simulink model "gm_Copy_of_uz_pmsm_model_9ph_21b_all_double"  (R2021b)
settings: Solver=FixedStepAuto  StartTime=0.0  StopTime=0.8  RelTol=1e-3
PreLoadFcn:
  | uz_pmsm_model_9ph_init_parameter
undefined symbols (not defined in the file or in its folder): a, b, c, friction_coefficient, inertia, k_i_d, k_i_q, k_p_d, k_p_q, Kpd, L_d, L_o1, L_o2, L_q, L_x1, L_x2, L_y1, L_y2, L_zero, polepair, psi_pm, R_1, static_friction_torque, Tnd, ts
libraries: hdlsllib x90, hdlmdlgenlib x17, slpidlib x2, simulink x2, spsAlphaBetaZerotodq0Lib x1, pid_lib x1, spsdq0toAlphaBetaZeroLib x1
(part 3 of 3)

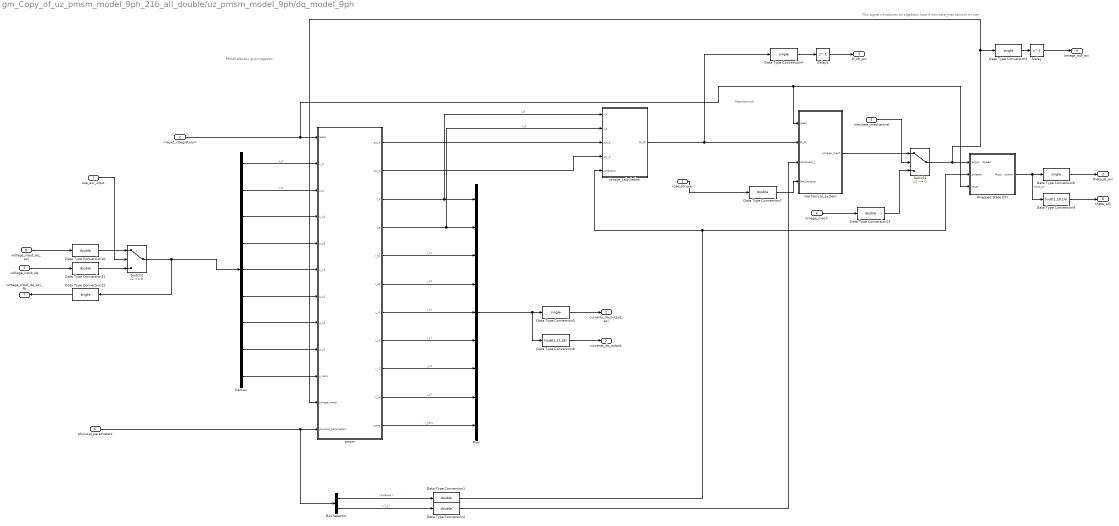
== system gm_Copy_of_uz_pmsm_model_9ph_21b_all_double/uz_pmsm_model_9ph/dq_model_9ph ==
  note: This signal introduces an algebraic loop if simulate_mechanical is true!
  note: PMSM electric and magentic
  note: Mechanical
  load_torque : Inport
  <reset_integrators> : Inport  Port=2
  simulate_mechanical : Inport  Port=3
  omega_mech : Inport  Port=4
  voltage_input_dq : Inport  Port=5
  physical_parameters : Inport  Port=6
  use_axi_input : Inport  Port=7
  voltage_input_dq_axi : Inport  Port=8
  Bus Selector : BusSelector  OutputSignals=polepair,1_J
  Data Type Conversion{1..2,7,10..11,13} (6 alike) : DataTypeConversion  OutDataTypeStr=double  RndMeth=Nearest
  Data Type Conversion{3..6,12} (5 alike) : DataTypeConversion  OutDataTypeStr=single  RndMeth=Nearest
  Data Type Conversion8 : DataTypeConversion  OutDataTypeStr=fixdt(1,27,18)  RndMeth=Nearest
  Data Type Conversion9 : DataTypeConversion  OutDataTypeStr=fixdt(1,18,14)  RndMeth=Nearest
  Delay : Delay  DelayLength=1
  Delay1 : Delay  DelayLength=1
  Demux : Demux  Outputs=9
  Mux : Mux  Inputs=9
  Switch1 : Switch  Criteria=u2 ~= 0
  Switch2 : Switch  Criteria=u2 ~= 0
  Wrapped State DTI : Subsystem
  mechanical_system : Subsystem
  pmsm : Subsystem
  torque_calculation : Subsystem
  currents_dq_output_axi : Outport
  theta_el_axi : Outport  Port=2
  M_Mi_axi : Outport  Port=3
  omega_out_axi : Outport  Port=4
  currents_dq_output : Outport  Port=5
  theta_el1 : Outport  Port=6
  voltage_input_dq_axi_fb : Outport  Port=7
  wires:
  Demux/5 -> pmsm/6(u_x1)
  Demux/7 -> pmsm/8(u_x2)
  Demux/3 -> pmsm/4(u_o1)
  pmsm/3(I_d) -> torque_calculation/1(I_d), Mux/1  "i_d"
  Demux/1 -> pmsm/2(u_d)  "u_d"
  pmsm/11(i_zero) -> Mux/9  "i_zero"
  pmsm/6(i_o2) -> Mux/4  "i_o2"
  Demux/4 -> pmsm/5(u_o2)
  Demux/2 -> pmsm/3(u_q)  "u_q"
  Demux/9 -> pmsm/10(u_zero)
  pmsm/9(i_x2) -> Mux/7  "i_x2"
  pmsm/7(i_x1) -> Mux/5  "i_x1"
  pmsm/10(i_y2) -> Mux/8  "i_y2"
  torque_calculation/1(M_Mi) -> Data Type Conversion4/1, mechanical_system/2(M_Mi)
  Demux/8 -> pmsm/9(u_y2)
  pmsm/1(psi_d) -> torque_calculation/3(psi_d)
  omega_mech/1 -> Data Type Conversion13/1
  pmsm/2(psi_q) -> torque_calculation/4(psi_q)
  simulate_mechanical/1 -> Switch1/2
  Demux/6 -> pmsm/7(u_y1)
  pmsm/5(i_o1) -> Mux/3  "i_o1"
  <reset_integrators>/1 -> Wrapped State DTI/3(reset), mechanical_system/1(reset), pmsm/1(reset)
  pmsm/4(I_q) -> torque_calculation/2(I_q), Mux/2  "i_q"
  mechanical_system/1(omega_mech) -> Switch1/1
  load_torque/1 -> Data Type Conversion7/1
  Switch1/1 -> pmsm/11(omega_mech), Data Type Conversion5/1, Wrapped State DTI/1(Angular Speed)
  pmsm/8(i_y1) -> Mux/6  "i_y1"
  Mux/1 -> Data Type Conversion8/1, Data Type Conversion3/1
  Bus Selector/1 -> Data Type Conversion1/1  "<polepair>"
  Bus Selector/2 -> Data Type Conversion2/1  "<1_J>"
  Delay/1 -> omega_out_axi/1
  Delay1/1 -> M_Mi_axi/1
  Switch2/1 -> Data Type Conversion12/1, Demux/1
  physical_parameters/1 -> Bus Selector/1, pmsm/12(physical_parameters)
  Data Type Conversion1/1 -> torque_calculation/5(polepairs), Wrapped State DTI/2(polepair)
  Data Type Conversion2/1 -> mechanical_system/3(reciprocal_J)
  Data Type Conversion3/1 -> currents_dq_output_axi/1
  Data Type Conversion4/1 -> Delay1/1
  Data Type Conversion5/1 -> Delay/1
  Data Type Conversion6/1 -> theta_el_axi/1
  Wrapped State DTI/1(Angular Position) -> Data Type Conversion9/1, Data Type Conversion6/1  "theta_el"
  Data Type Conversion7/1 -> mechanical_system/4(load_torque)
  Data Type Conversion9/1 -> theta_el1/1
  use_axi_input/1 -> Switch2/2
  voltage_input_dq/1 -> Data Type Conversion11/1
  voltage_input_dq_axi/1 -> Data Type Conversion10/1
  Data Type Conversion10/1 -> Switch2/1
  Data Type Conversion11/1 -> Switch2/3
  Data Type Conversion12/1 -> voltage_input_dq_axi_fb/1
  Data Type Conversion13/1 -> Switch1/3
  Data Type Conversion8/1 -> currents_dq_output/1

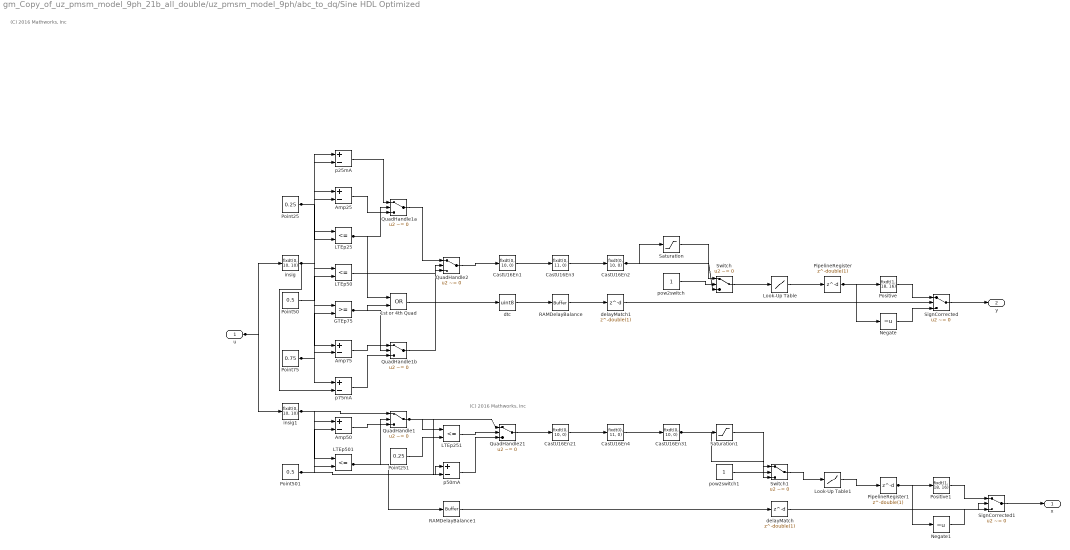
== system gm_Copy_of_uz_pmsm_model_9ph_21b_all_double/uz_pmsm_model_9ph/abc_to_dq/Sine HDL Optimized ==
  note: (C) 2016 Mathworks, Inc
  note: (C) 2016 Mathworks, Inc
  u : Inport  OutDataTypeStr=fixdt(1, 18, 16)  SampleTime=1e-08
  1st or 4th Quad : Logic  Operator=OR  AllPortsSameDT=off  OutDataTypeStr=boolean  SampleTime=1e-08
  Amp25 : Sum  Inputs=+-  AccumDataTypeStr=fixdt(1, 19, 18)  OutDataTypeStr=fixdt(1, 19, 18)  SampleTime=1e-08
  Amp50 : Sum  Inputs=+-  AccumDataTypeStr=fixdt(1, 19, 18)  OutDataTypeStr=fixdt(1, 19, 18)  SampleTime=1e-08
  Amp75 : Sum  Inputs=+-  AccumDataTypeStr=fixdt(1, 19, 18)  OutDataTypeStr=fixdt(1, 19, 18)  SampleTime=1e-08
  CastU16En1 : DataTypeConversion  OutDataTypeStr=fixdt(0, 10, 0)  ConvertRealWorld=Stored Integer (SI)  SampleTime=1e-08
  CastU16En2 : DataTypeConversion  OutDataTypeStr=fixdt(0, 10, 0)  ConvertRealWorld=Stored Integer (SI)  SampleTime=1e-08  SaturateOnIntegerOverflow=on
  CastU16En21 : DataTypeConversion  OutDataTypeStr=fixdt(0, 10, 0)  ConvertRealWorld=Stored Integer (SI)  SampleTime=1e-08
  CastU16En3 : DataTypeConversion  OutDataTypeStr=fixdt(0, 11, 0)  SampleTime=1e-08
  CastU16En31 : DataTypeConversion  OutDataTypeStr=fixdt(0, 10, 0)  ConvertRealWorld=Stored Integer (SI)  SampleTime=1e-08  SaturateOnIntegerOverflow=on
  CastU16En4 : DataTypeConversion  OutDataTypeStr=fixdt(0, 11, 0)  SampleTime=1e-08
  GTEp75 : RelationalOperator  OutDataTypeStr=boolean  SampleTime=1e-08  RndMeth=Nearest
  LTEp{25,50,251,501} (4 alike) : RelationalOperator  Operator=<=  OutDataTypeStr=boolean  SampleTime=1e-08  RndMeth=Nearest
  Look-Up Table : Lookup_n-D  NumberOfTableDimensions=1  BreakpointsForDimension1="fi(\"numerictype\",numerictype(0,10,0),\"fimath\",fimath(\"RoundingMethod\", \"Floor\",\"OverflowAction\", \"Wrap\",\"ProductMode\",\"FullPrecision\",\"SumMode\",\"FullPrecision\"),\"Value\",\"[0 1 2 3 4 5 6 7 8 9 10 11 12 13 14 15 16 17 18 19 20 21 22 23 24 25 26 27 28 29 30 31 32 33 34 35 36 37 38 39 40 41 42 43 44 45 46 47 48 49 50 51 52 53 54 55 56 57 58 59 60 61 62 63 64 65 66 67 68 69 70 71 72 73 74 75 76 77 78 79 80 81 82 83 84 85 86 87 88 89 90 91 92 93 94 95 96 97 98 99 100 101 102 103 104 105 106 107 108 109 110 111 112 113 114 115 116 117 118 119 120 121 122 123 124 125 126 127 128 129 130 131 132 133 134 135 136 137 138 139 140 141 142 143 144 145 146 147 148 149 150 151 152 153 154 155 156 157 158 159 160 161 162 163 164 165 166 167 168 169 170 171 172 173 174 175 176 177 178 179 180 181 182 183 184 185 186 187 188 189 190 191 192 193 194 195 196 197 198 199 200 201 202 203 204 205 206 207 208 209 210 211 212 213 214 215 216 217 218 219 220 221 222 223 224 225 226 227 228 229 230 231 232 233 234 235 236 237 238 239 240 241 242 243 244 245 246 247 248 249 250 251 252 253 254 255]\")"  Table="reshape(fi(\"numerictype\",numerictype(1,18,16),\"fimath\",fimath(\"RoundingMethod\", \"Floor\",\"OverflowAction\", \"Wrap\",\"ProductMode\",\"FullPrecision\",\"SumMode\",\"FullPrecision\"),\"Value\",\"[0;0.006134033203125;0.01226806640625;0.018402099609375;0.0245361328125;0.030670166015625;0.03680419921875;0.042938232421875;0.049072265625;0.0551910400390625;0.0613250732421875;0.06744384765625;0.0735626220703125;0.079681396484375;0.0858001708984375;0.0919036865234375;0.0980224609375;0.1041259765625;0.1102294921875;0.1163177490234375;0.122406005859375;0.1284942626953125;0.13458251953125;0.140655517578125;0.146728515625;0.152801513671875;0.1588592529296875;0.1649169921875;0.17095947265625;0.177001953125;0.18304443359375;0.1890716552734375;0.1950836181640625;0.20111083984375;0.2071075439453125;0.213104248046875;0.2191009521484375;0.2250823974609375;0.2310638427734375;0.237030029296875;0.24298095703125;0.248931884765625;0.2548675537109375;0.2607879638671875;0.2667083740234375;0.2726287841796875;0.2785186767578125;0.2844085693359375;0.290283203125;0.2961578369140625;0.302001953125;0.3078460693359375;0.3136749267578125;0.3195037841796875;0.3253173828125;0.3311004638671875;0.336883544921875;0.3426666259765625;0.348419189453125;0.354156494140625;0.359893798828125;0.3656158447265625;0.3713226318359375;0.37701416015625;0.3826904296875;0.3883514404296875;0.3939971923828125;0.399627685546875;0.405242919921875;0.4108428955078125;0.4164276123046875;0.4219970703125;0.42755126953125;0.4330902099609375;0.4386138916015625;0.444122314453125;0.449615478515625;0.455078125;0.460540771484375;0.465972900390625;0.4713897705078125;0.476806640625;0.482177734375;0.487548828125;0.4929046630859375;0.49822998046875;0.5035400390625;0.5088348388671875;0.51409912109375;0.5193634033203125;0.52459716796875;0.5298004150390625;0.535003662109375;0.5401763916015625;0.545318603515625;0.5504608154296875;0.555572509765625;0.5606689453125;0.56573486328125;0.5707855224609375;0.5758056640625;0.580810546875;0.5858001708984375;0.59075927734375;0.595703125;0.600616455078125;0.6055145263671875;0.610382080078125;0.615234375;0.62005615234375;0.6248626708984375;0.629638671875;0.6343994140625;0.639129638671875;0.643829345703125;0.6485137939453125;0.653167724609375;0.657806396484375;0.66241455078125;0.6670074462890625;0.6715545654296875;0.67608642578125;0.68060302734375;0.685089111328125;0.689544677734375;0.6939697265625;0.6983795166015625;0.7027587890625;0.7071075439453125;0.71142578125;0.715728759765625;0.720001220703125;0.7242431640625;0.7284698486328125;0.7326507568359375;0.73681640625;0.7409515380859375;0.74505615234375;0.7491302490234375;0.7531890869140625;0.7572021484375;0.761199951171875;0.765167236328125;0.76910400390625;0.77301025390625;0.776885986328125;0.780731201171875;0.7845611572265625;0.7883453369140625;0.7920989990234375;0.79583740234375;0.799530029296875;0.8032073974609375;0.806854248046875;0.810455322265625;0.8140411376953125;0.8175811767578125;0.82110595703125;0.8245849609375;0.8280487060546875;0.8314666748046875;0.834869384765625;0.838226318359375;0.841552734375;0.8448486328125;0.848114013671875;0.851348876953125;0.85455322265625;0.85772705078125;0.860870361328125;0.8639678955078125;0.8670501708984375;0.870086669921875;0.8730926513671875;0.876068115234375;0.8790130615234375;0.881927490234375;0.884796142578125;0.88763427734375;0.89044189453125;0.893218994140625;0.895965576171875;0.898681640625;0.9013519287109375;0.90399169921875;0.9066009521484375;0.9091644287109375;0.911712646484375;0.914215087890625;0.9166717529296875;0.9191131591796875;0.9215087890625;0.9238739013671875;0.92620849609375;0.9285125732421875;0.9307708740234375;0.9329986572265625;0.9351806640625;0.9373321533203125;0.939453125;0.9415435791015625;0.9435882568359375;0.9456024169921875;0.9475860595703125;0.94952392578125;0.9514312744140625;0.95330810546875;0.95513916015625;0.956939697265625;0.958709716796875;0.9604339599609375;0.962127685546875;0.963775634765625;0.96539306640625;0.96697998046875;0.9685211181640625;0.97003173828125;0.97149658203125;0.9729461669921875;0.974334716796875;0.9757080078125;0.9770355224609375;0.9783172607421875;0.9795684814453125;0.9807891845703125;0.981964111328125 ...(+541 chars)]\"), [1  256])"  InterpMethod=Flat  ExtrapMethod=Clip  DiagnosticForOutOfRangeInput=Error  SampleTime=1e-08  OutDataTypeStr=fixdt(1, 18, 16)  InputSameDT=on
  Look-Up Table1 : Lookup_n-D  NumberOfTableDimensions=1  BreakpointsForDimension1="fi(\"numerictype\",numerictype(0,10,0),\"fimath\",fimath(\"RoundingMethod\", \"Floor\",\"OverflowAction\", \"Wrap\",\"ProductMode\",\"FullPrecision\",\"SumMode\",\"FullPrecision\"),\"Value\",\"[0 1 2 3 4 5 6 7 8 9 10 11 12 13 14 15 16 17 18 19 20 21 22 23 24 25 26 27 28 29 30 31 32 33 34 35 36 37 38 39 40 41 42 43 44 45 46 47 48 49 50 51 52 53 54 55 56 57 58 59 60 61 62 63 64 65 66 67 68 69 70 71 72 73 74 75 76 77 78 79 80 81 82 83 84 85 86 87 88 89 90 91 92 93 94 95 96 97 98 99 100 101 102 103 104 105 106 107 108 109 110 111 112 113 114 115 116 117 118 119 120 121 122 123 124 125 126 127 128 129 130 131 132 133 134 135 136 137 138 139 140 141 142 143 144 145 146 147 148 149 150 151 152 153 154 155 156 157 158 159 160 161 162 163 164 165 166 167 168 169 170 171 172 173 174 175 176 177 178 179 180 181 182 183 184 185 186 187 188 189 190 191 192 193 194 195 196 197 198 199 200 201 202 203 204 205 206 207 208 209 210 211 212 213 214 215 216 217 218 219 220 221 222 223 224 225 226 227 228 229 230 231 232 233 234 235 236 237 238 239 240 241 242 243 244 245 246 247 248 249 250 251 252 253 254 255]\")"  Table="reshape(fi(\"numerictype\",numerictype(1,18,16),\"fimath\",fimath(\"RoundingMethod\", \"Floor\",\"OverflowAction\", \"Wrap\",\"ProductMode\",\"FullPrecision\",\"SumMode\",\"FullPrecision\"),\"Value\",\"[0;0.006134033203125;0.01226806640625;0.018402099609375;0.0245361328125;0.030670166015625;0.03680419921875;0.042938232421875;0.049072265625;0.0551910400390625;0.0613250732421875;0.06744384765625;0.0735626220703125;0.079681396484375;0.0858001708984375;0.0919036865234375;0.0980224609375;0.1041259765625;0.1102294921875;0.1163177490234375;0.122406005859375;0.1284942626953125;0.13458251953125;0.140655517578125;0.146728515625;0.152801513671875;0.1588592529296875;0.1649169921875;0.17095947265625;0.177001953125;0.18304443359375;0.1890716552734375;0.1950836181640625;0.20111083984375;0.2071075439453125;0.213104248046875;0.2191009521484375;0.2250823974609375;0.2310638427734375;0.237030029296875;0.24298095703125;0.248931884765625;0.2548675537109375;0.2607879638671875;0.2667083740234375;0.2726287841796875;0.2785186767578125;0.2844085693359375;0.290283203125;0.2961578369140625;0.302001953125;0.3078460693359375;0.3136749267578125;0.3195037841796875;0.3253173828125;0.3311004638671875;0.336883544921875;0.3426666259765625;0.348419189453125;0.354156494140625;0.359893798828125;0.3656158447265625;0.3713226318359375;0.37701416015625;0.3826904296875;0.3883514404296875;0.3939971923828125;0.399627685546875;0.405242919921875;0.4108428955078125;0.4164276123046875;0.4219970703125;0.42755126953125;0.4330902099609375;0.4386138916015625;0.444122314453125;0.449615478515625;0.455078125;0.460540771484375;0.465972900390625;0.4713897705078125;0.476806640625;0.482177734375;0.487548828125;0.4929046630859375;0.49822998046875;0.5035400390625;0.5088348388671875;0.51409912109375;0.5193634033203125;0.52459716796875;0.5298004150390625;0.535003662109375;0.5401763916015625;0.545318603515625;0.5504608154296875;0.555572509765625;0.5606689453125;0.56573486328125;0.5707855224609375;0.5758056640625;0.580810546875;0.5858001708984375;0.59075927734375;0.595703125;0.600616455078125;0.6055145263671875;0.610382080078125;0.615234375;0.62005615234375;0.6248626708984375;0.629638671875;0.6343994140625;0.639129638671875;0.643829345703125;0.6485137939453125;0.653167724609375;0.657806396484375;0.66241455078125;0.6670074462890625;0.6715545654296875;0.67608642578125;0.68060302734375;0.685089111328125;0.689544677734375;0.6939697265625;0.6983795166015625;0.7027587890625;0.7071075439453125;0.71142578125;0.715728759765625;0.720001220703125;0.7242431640625;0.7284698486328125;0.7326507568359375;0.73681640625;0.7409515380859375;0.74505615234375;0.7491302490234375;0.7531890869140625;0.7572021484375;0.761199951171875;0.765167236328125;0.76910400390625;0.77301025390625;0.776885986328125;0.780731201171875;0.7845611572265625;0.7883453369140625;0.7920989990234375;0.79583740234375;0.799530029296875;0.8032073974609375;0.806854248046875;0.810455322265625;0.8140411376953125;0.8175811767578125;0.82110595703125;0.8245849609375;0.8280487060546875;0.8314666748046875;0.834869384765625;0.838226318359375;0.841552734375;0.8448486328125;0.848114013671875;0.851348876953125;0.85455322265625;0.85772705078125;0.860870361328125;0.8639678955078125;0.8670501708984375;0.870086669921875;0.8730926513671875;0.876068115234375;0.8790130615234375;0.881927490234375;0.884796142578125;0.88763427734375;0.89044189453125;0.893218994140625;0.895965576171875;0.898681640625;0.9013519287109375;0.90399169921875;0.9066009521484375;0.9091644287109375;0.911712646484375;0.914215087890625;0.9166717529296875;0.9191131591796875;0.9215087890625;0.9238739013671875;0.92620849609375;0.9285125732421875;0.9307708740234375;0.9329986572265625;0.9351806640625;0.9373321533203125;0.939453125;0.9415435791015625;0.9435882568359375;0.9456024169921875;0.9475860595703125;0.94952392578125;0.9514312744140625;0.95330810546875;0.95513916015625;0.956939697265625;0.958709716796875;0.9604339599609375;0.962127685546875;0.963775634765625;0.96539306640625;0.96697998046875;0.9685211181640625;0.97003173828125;0.97149658203125;0.9729461669921875;0.974334716796875;0.9757080078125;0.9770355224609375;0.9783172607421875;0.9795684814453125;0.9807891845703125;0.981964111328125 ...(+541 chars)]\"), [1  256])"  InterpMethod=Flat  ExtrapMethod=Clip  DiagnosticForOutOfRangeInput=Error  SampleTime=1e-08  OutDataTypeStr=fixdt(1, 18, 16)  InputSameDT=on
  Negate : UnaryMinus  SampleTime=1e-08
  Negate1 : UnaryMinus  SampleTime=1e-08
  PipelineRegister : Delay  DelayLength=double(1)  InitialCondition=0  SampleTime=1e-08
  PipelineRegister1 : Delay  DelayLength=double(1)  InitialCondition=0  SampleTime=1e-08
  Point25 : Constant  Value=0.25  OutDataTypeStr=fixdt(0, 18, 18)  SampleTime=1e-08
  Point251 : Constant  Value=0.25  OutDataTypeStr=fixdt(0, 18, 18)  SampleTime=1e-08
  Point50 : Constant  Value=0.5  OutDataTypeStr=fixdt(0, 18, 18)  SampleTime=1e-08
  Point501 : Constant  Value=0.5  OutDataTypeStr=fixdt(0, 18, 18)  SampleTime=1e-08
  Point75 : Constant  Value=0.75  OutDataTypeStr=fixdt(0, 18, 18)  SampleTime=1e-08
  Positive : DataTypeConversion  OutDataTypeStr=fixdt(1, 18, 16)  SampleTime=1e-08
  Positive1 : DataTypeConversion  OutDataTypeStr=fixdt(1, 18, 16)  SampleTime=1e-08
  QuadHandle1 : Switch  Criteria=u2 ~= 0  Threshold=double(0)  OutDataTypeStr=fixdt(1, 19, 18)  SampleTime=1e-08
  QuadHandle1a : Switch  Criteria=u2 ~= 0  Threshold=double(0)  OutDataTypeStr=fixdt(1, 19, 18)  SampleTime=1e-08
  QuadHandle1b : Switch  Criteria=u2 ~= 0  Threshold=double(0)  OutDataTypeStr=fixdt(1, 19, 18)  SampleTime=1e-08
  QuadHandle2 : Switch  Criteria=u2 ~= 0  Threshold=double(0)  OutDataTypeStr=fixdt(0, 10, 10)  SampleTime=1e-08  SaturateOnIntegerOverflow=on
  QuadHandle21 : Switch  Criteria=u2 ~= 0  Threshold=double(0)  OutDataTypeStr=fixdt(0, 10, 10)  SampleTime=1e-08
  RAMDelayBalance : hdlmdlgenlib/Buffer
      settings: SourceProductBaseCode=SL
  RAMDelayBalance1 : hdlmdlgenlib/Buffer
      settings: SourceProductBaseCode=SL
  Saturation : Saturate  UpperLimit="fi(0,0,10,0,\"hex\",\"0ff\")"  LowerLimit="fi(0,0,10,0,\"hex\",\"000\")"  SampleTime=1e-08  OutDataTypeStr=fixdt(0, 10, 0)
  Saturation1 : Saturate  UpperLimit="fi(0,0,10,0,\"hex\",\"0ff\")"  LowerLimit="fi(0,0,10,0,\"hex\",\"000\")"  SampleTime=1e-08  OutDataTypeStr=fixdt(0, 10, 0)
  SignCorrected : Switch  Criteria=u2 ~= 0  Threshold=double(0)  OutDataTypeStr=fixdt(1, 18, 16)  SampleTime=1e-08
  SignCorrected1 : Switch  Criteria=u2 ~= 0  Threshold=double(0)  OutDataTypeStr=fixdt(1, 18, 16)  SampleTime=1e-08
  Switch : Switch  Criteria=u2 ~= 0  Threshold=double(0)  OutDataTypeStr=fixdt(0, 10, 0)  SampleTime=1e-08
  Switch1 : Switch  Criteria=u2 ~= 0  Threshold=double(0)  OutDataTypeStr=fixdt(0, 10, 0)  SampleTime=1e-08
  delayMatch : Delay  DelayLength=double(1)  InitialCondition=0  SampleTime=1e-08
  delayMatch1 : Delay  DelayLength=double(1)  InitialCondition=0  SampleTime=1e-08
  dtc : DataTypeConversion  OutDataTypeStr=uint8  SampleTime=1e-08
  insig : DataTypeConversion  OutDataTypeStr=fixdt(0, 10, 10)  SampleTime=1e-08
  insig1 : DataTypeConversion  OutDataTypeStr=fixdt(0, 10, 10)  SampleTime=1e-08
  p25mA : Sum  Inputs=+-  AccumDataTypeStr=fixdt(1, 19, 18)  OutDataTypeStr=fixdt(1, 19, 18)  SampleTime=1e-08
  p50mA : Sum  Inputs=+-  AccumDataTypeStr=fixdt(1, 20, 18)  OutDataTypeStr=fixdt(1, 20, 18)  SampleTime=1e-08
  p75mA : Sum  Inputs=+-  AccumDataTypeStr=fixdt(1, 19, 18)  OutDataTypeStr=fixdt(1, 19, 18)  SampleTime=1e-08
  pow2switch : Constant  OutDataTypeStr=boolean  SampleTime=1e-08
  pow2switch1 : Constant  OutDataTypeStr=boolean  SampleTime=1e-08
  x : Outport  SampleTime=1e-08
  y : Outport  Port=2  SampleTime=1e-08
  wires:
  dtc/1 -> RAMDelayBalance/1
  Amp25/1 -> QuadHandle1a/3
  Amp75/1 -> QuadHandle1b/1
  CastU16En1/1 -> CastU16En3/1
  CastU16En2/1 -> Switch/3, Saturation/1
  CastU16En3/1 -> CastU16En2/1
  GTEp75/1 -> QuadHandle1b/2, 1st or 4th Quad/2
  LTEp25/1 -> QuadHandle1a/2, 1st or 4th Quad/1
  LTEp50/1 -> QuadHandle2/2
  PipelineRegister/1 -> Positive/1, Negate/1
  Negate/1 -> SignCorrected/3
  Point25/1 -> p25mA/1, LTEp25/2, Amp25/2
  Point50/1 -> LTEp50/2
  Point75/1 -> p75mA/1, GTEp75/2, Amp75/2
  Positive/1 -> SignCorrected/1
  QuadHandle1a/1 -> QuadHandle2/1
  QuadHandle1b/1 -> QuadHandle2/3
  QuadHandle2/1 -> CastU16En1/1
  delayMatch1/1 -> SignCorrected/2
  Saturation/1 -> Switch/1
  SignCorrected/1 -> y/1
  Switch/1 -> Look-Up Table/1
  insig/1 -> p75mA/2, p25mA/2, LTEp50/1, LTEp25/1, GTEp75/1, Amp75/1, Amp25/1
  p25mA/1 -> QuadHandle1a/1
  p75mA/1 -> QuadHandle1b/3
  pow2switch/1 -> Switch/2
  Amp50/1 -> QuadHandle1/3
  CastU16En21/1 -> CastU16En4/1
  CastU16En31/1 -> Switch1/3, Saturation1/1
  CastU16En4/1 -> CastU16En31/1
  LTEp251/1 -> QuadHandle21/2
  LTEp501/1 -> QuadHandle1/2, RAMDelayBalance1/1
  PipelineRegister1/1 -> Positive1/1, Negate1/1
  Negate1/1 -> SignCorrected1/3
  Point251/1 -> LTEp251/2
  Point501/1 -> p50mA/1, LTEp501/2, Amp50/2
  Positive1/1 -> SignCorrected1/1
  QuadHandle1/1 -> p50mA/2, QuadHandle21/1, LTEp251/1
  QuadHandle21/1 -> CastU16En21/1
  delayMatch/1 -> SignCorrected1/2
  Saturation1/1 -> Switch1/1
  SignCorrected1/1 -> x/1
  Switch1/1 -> Look-Up Table1/1
  insig1/1 -> QuadHandle1/1, LTEp501/1, Amp50/1
  p50mA/1 -> QuadHandle21/3
  pow2switch1/1 -> Switch1/2
  1st or 4th Quad/1 -> dtc/1
  RAMDelayBalance1/1 -> delayMatch/1
  RAMDelayBalance/1 -> delayMatch1/1
  u/1 -> insig1/1, insig/1
  Look-Up Table/1 -> PipelineRegister/1
  Look-Up Table1/1 -> PipelineRegister1/1

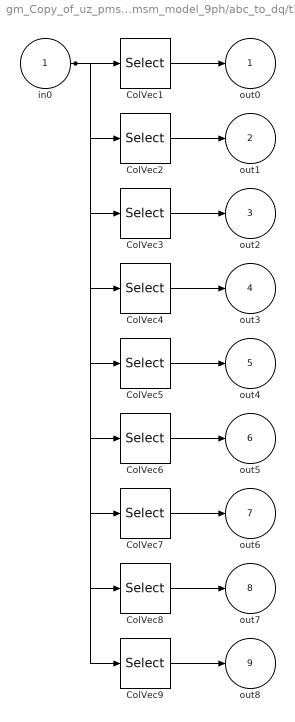
== system gm_Copy_of_uz_pmsm_model_9ph_21b_all_double/uz_pmsm_model_9ph/abc_to_dq/t19 ==
  in0 : Inport
  ColVec1 : Selector  NumberOfDimensions=2  IndexOptions=Select all,Index vector (dialog)  Indices=1,1  OutputSizes=1,1
  ColVec2 : Selector  NumberOfDimensions=2  IndexOptions=Select all,Index vector (dialog)  Indices=1,2  OutputSizes=1,1
  ColVec3 : Selector  NumberOfDimensions=2  IndexOptions=Select all,Index vector (dialog)  Indices=1,3  OutputSizes=1,1
  ColVec4 : Selector  NumberOfDimensions=2  IndexOptions=Select all,Index vector (dialog)  Indices=1,4  OutputSizes=1,1
  ColVec5 : Selector  NumberOfDimensions=2  IndexOptions=Select all,Index vector (dialog)  Indices=1,5  OutputSizes=1,1
  ColVec6 : Selector  NumberOfDimensions=2  IndexOptions=Select all,Index vector (dialog)  Indices=1,6  OutputSizes=1,1
  ColVec7 : Selector  NumberOfDimensions=2  IndexOptions=Select all,Index vector (dialog)  Indices=1,7  OutputSizes=1,1
  ColVec8 : Selector  NumberOfDimensions=2  IndexOptions=Select all,Index vector (dialog)  Indices=1,8  OutputSizes=1,1
  ColVec9 : Selector  NumberOfDimensions=2  IndexOptions=Select all,Index vector (dialog)  Indices=1,9  OutputSizes=1,1
  out0 : Outport
  out1 : Outport  Port=2
  out2 : Outport  Port=3
  out3 : Outport  Port=4
  out4 : Outport  Port=5
  out5 : Outport  Port=6
  out6 : Outport  Port=7
  out7 : Outport  Port=8
  out8 : Outport  Port=9
  wires:
  in0/1 -> ColVec1/1, ColVec2/1, ColVec3/1, ColVec4/1, ColVec5/1, ColVec6/1, ColVec7/1, ColVec8/1, ColVec9/1
  ColVec1/1 -> out0/1
  ColVec2/1 -> out1/1
  ColVec3/1 -> out2/1
  ColVec4/1 -> out3/1
  ColVec5/1 -> out4/1
  ColVec6/1 -> out5/1
  ColVec7/1 -> out6/1
  ColVec8/1 -> out7/1
  ColVec9/1 -> out8/1

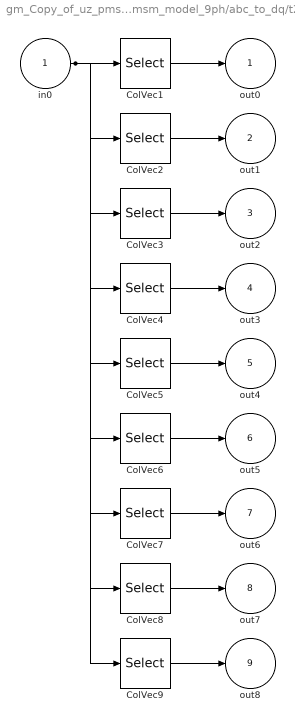
== system gm_Copy_of_uz_pmsm_model_9ph_21b_all_double/uz_pmsm_model_9ph/abc_to_dq/t23 ==
  in0 : Inport
  ColVec1 : Selector  NumberOfDimensions=2  IndexOptions=Select all,Index vector (dialog)  Indices=1,1  OutputSizes=1,1
  ColVec2 : Selector  NumberOfDimensions=2  IndexOptions=Select all,Index vector (dialog)  Indices=1,2  OutputSizes=1,1
  ColVec3 : Selector  NumberOfDimensions=2  IndexOptions=Select all,Index vector (dialog)  Indices=1,3  OutputSizes=1,1
  ColVec4 : Selector  NumberOfDimensions=2  IndexOptions=Select all,Index vector (dialog)  Indices=1,4  OutputSizes=1,1
  ColVec5 : Selector  NumberOfDimensions=2  IndexOptions=Select all,Index vector (dialog)  Indices=1,5  OutputSizes=1,1
  ColVec6 : Selector  NumberOfDimensions=2  IndexOptions=Select all,Index vector (dialog)  Indices=1,6  OutputSizes=1,1
  ColVec7 : Selector  NumberOfDimensions=2  IndexOptions=Select all,Index vector (dialog)  Indices=1,7  OutputSizes=1,1
  ColVec8 : Selector  NumberOfDimensions=2  IndexOptions=Select all,Index vector (dialog)  Indices=1,8  OutputSizes=1,1
  ColVec9 : Selector  NumberOfDimensions=2  IndexOptions=Select all,Index vector (dialog)  Indices=1,9  OutputSizes=1,1
  out0 : Outport
  out1 : Outport  Port=2
  out2 : Outport  Port=3
  out3 : Outport  Port=4
  out4 : Outport  Port=5
  out5 : Outport  Port=6
  out6 : Outport  Port=7
  out7 : Outport  Port=8
  out8 : Outport  Port=9
  wires:
  in0/1 -> ColVec1/1, ColVec2/1, ColVec3/1, ColVec4/1, ColVec5/1, ColVec6/1, ColVec7/1, ColVec8/1, ColVec9/1
  ColVec1/1 -> out0/1
  ColVec2/1 -> out1/1
  ColVec3/1 -> out2/1
  ColVec4/1 -> out3/1
  ColVec5/1 -> out4/1
  ColVec6/1 -> out5/1
  ColVec7/1 -> out6/1
  ColVec8/1 -> out7/1
  ColVec9/1 -> out8/1

== system gm_Copy_of_uz_pmsm_model_9ph_21b_all_double/uz_pmsm_model_9ph/dq_model_9ph/Wrapped State DTI ==
  note: https://de.mathworks.com/help/releases/R2021a/hdlcoder/ug/troubleshoot-generate-implementation-model-from-simscape-pmsm.html?searchHighlight=troubleshoot-generate-implementation-model-from-simscape-pmsm&s_tid=doc_srchtitle
  Angular Speed : Inport
  polepair : Inport  Port=2
  reset : Inport  Port=3
  Compare To Constant : simulink/Logic and Bit Operations/Compare To Constant  relop=>=  const=single(pi)  OutDataTypeStr=boolean
  Compare To Constant1 : simulink/Logic and Bit Operations/Compare To Constant  relop=<  const=single(-pi)  OutDataTypeStr=boolean
  Constant : Constant  Value=double(2*pi)  SampleTime=-1
  Delay1 : Delay  DelayLength=1  ExternalReset=Level
      settings: InputPortMap=u0,r5
  Gain : Gain  Gain=ts
  Product : Product
  Sum : Sum  Inputs=|++
  Sum1 : Sum  Inputs=|-+
  Sum2 : Sum  Inputs=|++
  Switch : Switch  Criteria=u2 > Threshold
  Switch1 : Switch  Criteria=u2 > Threshold
  Angular Position : Outport
  wires:
  Compare To Constant1/1 -> Switch1/2
  Delay1/1 -> Sum/1, Angular Position/1
  Constant/1 -> Sum2/1, Sum1/1
  Sum2/1 -> Switch1/1
  Switch1/1 -> Delay1/1  "Angular Position"
  Switch/1 -> Sum2/2, Compare To Constant1/1, Switch1/3
  Compare To Constant/1 -> Switch/2
  Sum/1 -> Compare To Constant/1, Sum1/2, Switch/3
  Sum1/1 -> Switch/1
  Gain/1 -> Sum/2
  reset/1 -> Delay1/2
  Product/1 -> Gain/1
  Angular Speed/1 -> Product/1
  polepair/1 -> Product/2

== system gm_Copy_of_uz_pmsm_model_9ph_21b_all_double/uz_pmsm_model_9ph/dq_model_9ph/mechanical_system ==
  note: load torque negative!!!
  note: This delay breaks the algebraic loop between mechanical and electrical system.
      | Introduces a delay of 500ns.
  reset : Inport
  M_Mi : Inport  Port=2
  reciprocal_J : Inport  Port=3
  load_torque : Inport  Port=4
  Delay : Delay  DelayLength=1
  Product11 : Product
  Sum1 : Sum  Inputs=|++
  integrator : Subsystem
  omega_mech : Outport
  wires:
  reciprocal_J/1 -> Product11/1
  Sum1/1 -> Product11/2
  load_torque/1 -> Sum1/2
  M_Mi/1 -> Delay/1
  Delay/1 -> Sum1/1
  integrator/1(outt) -> omega_mech/1
  Product11/1 -> integrator/1(in)
  reset/1 -> integrator/2(reset)

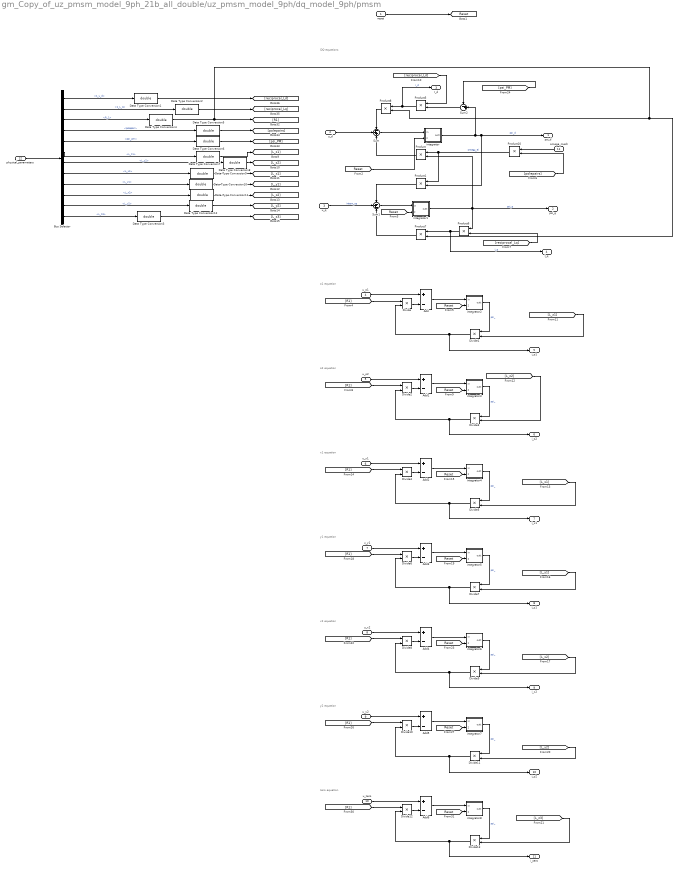
== system gm_Copy_of_uz_pmsm_model_9ph_21b_all_double/uz_pmsm_model_9ph/dq_model_9ph/pmsm ==
  note: o1 equation
  note: DQ equations
  note: o2 equation
  note: x1 equation
  note: y1 equation
  note: x2 equation
  note: y2 equation
  note: zero equation
  reset : Inport
  u_d : Inport  Port=2
  u_q : Inport  Port=3
  u_o1 : Inport  Port=4
  u_o2 : Inport  Port=5
  u_x1 : Inport  Port=6
  u_y1 : Inport  Port=7
  u_x2 : Inport  Port=8
  u_y2 : Inport  Port=9
  u_zero : Inport  Port=10
  omega_mech : Inport  Port=11
  physical_parameters : Inport  Port=12
  Add{,1..6} (7 alike) : Sum  Inputs=+-
  Bus Selector : BusSelector  OutputSignals=1_L_d,1_L_q,R_1,polepair,psi_pm,L_z1,L_z2,L_x1,L_y1,L_x2,L_y2,L_z3
  Data Type Conversion{1..12} (12 alike) : DataTypeConversion  OutDataTypeStr=double  RndMeth=Nearest
  Divide{,1..13} (14 alike) : Product  Inputs=**
  Product{,1,5..8,10} (7 alike) : Product
  Sum : Sum  Inputs=-++
  Sum1 : Sum  Inputs=-+-
  Sum2 : Sum  Inputs=-+|
  integrator : Subsystem
  integrator1 : Subsystem
  integrator2 : Subsystem
  integrator3 : Subsystem
  integrator4 : Subsystem
  integrator5 : Subsystem
  integrator6 : Subsystem
  integrator7 : Subsystem
  integrator8 : Subsystem
  psi_d : Outport
  psi_q : Outport  Port=2
  I_d : Outport  Port=3
  I_q : Outport  Port=4
  i_o1 : Outport  Port=5
  i_o2 : Outport  Port=6
  i_x1 : Outport  Port=7
  i_y1 : Outport  Port=8
  i_x2 : Outport  Port=9
  i_y2 : Outport  Port=10
  i_zero : Outport  Port=11
  tag scope: Reset=global
  wires:
  omega_mech/1 -> Product10/1
  u_q/1 -> Sum1/2  "intern_uq"
  Product/1 -> Sum/3
  Product5/1 -> I_d/1, Product8/1  "I_d"
  [reciprocal_Ld] -> Product5/1
  integrator1/1(outt) -> psi_q/1, Product/2, Product6/1  "psi_q"
  Product1/1 -> Sum1/1
  [psi_PM] -> Sum2/1
  Product6/1 -> I_q/1, Product7/1  "I_q"
  Product10/1 -> Product1/1, Product/1  "omega_el"
  integrator/1(outt) -> Sum2/2, psi_d/1, Product1/2  "psi_d"
  Sum2/1 -> Product5/2
  Product8/1 -> Sum/1
  [reciprocal_Lq] -> Product6/2
  Product7/1 -> Sum1/3
  reset/1 -> [Reset]
  [Reset] -> integrator/2(reset)
  [Reset] -> integrator1/2(reset)
  [Reset] -> integrator2/2(reset)
  [L_z1] -> Divide1/2
  u_o1/1 -> Add/1
  Divide1/1 -> i_o1/1, Divide/2
  Divide/1 -> Add/2
  [R1] -> Divide/1
  integrator2/1(outt) -> Divide1/1  "psi_"
  integrator3/1(outt) -> Divide3/1  "psi_"
  [R1] -> Divide2/1
  Divide2/1 -> Add1/2
  Divide3/1 -> i_o2/1, Divide2/2
  u_o2/1 -> Add1/1
  [L_z2] -> Divide3/2
  [Reset] -> integrator3/2(reset)
  [Reset] -> integrator4/2(reset)
  u_x1/1 -> Add2/1
  Divide5/1 -> i_x1/1, Divide4/2
  Divide4/1 -> Add2/2
  [R1] -> Divide4/1
  integrator4/1(outt) -> Divide5/1  "psi_"
  integrator5/1(outt) -> Divide7/1  "psi_"
  [R1] -> Divide6/1
  Divide6/1 -> Add3/2
  Divide7/1 -> i_y1/1, Divide6/2
  u_y1/1 -> Add3/1
  [Reset] -> integrator5/2(reset)
  [Reset] -> integrator6/2(reset)
  u_x2/1 -> Add4/1
  Divide9/1 -> i_x2/1, Divide8/2
  Divide8/1 -> Add4/2
  [R1] -> Divide8/1
  integrator6/1(outt) -> Divide9/1  "psi_"
  integrator7/1(outt) -> Divide11/1  "psi_"
  [R1] -> Divide10/1
  Divide10/1 -> Add5/2
  Divide11/1 -> i_y2/1, Divide10/2
  u_y2/1 -> Add5/1
  [Reset] -> integrator7/2(reset)
  [Reset] -> integrator8/2(reset)
  u_zero/1 -> Add6/1
  Divide13/1 -> i_zero/1, Divide12/2
  Divide12/1 -> Add6/2
  [R1] -> Divide12/1
  integrator8/1(outt) -> Divide13/1  "psi_"
  Bus Selector/1 -> Data Type Conversion1/1  "<1_L_d>"
  Bus Selector/4 -> Data Type Conversion5/1  "<polepair>"
  Bus Selector/8 -> Data Type Conversion9/1  "<L_x1>"
  Bus Selector/2 -> Data Type Conversion2/1  "<1_L_q>"
  Bus Selector/5 -> Data Type Conversion6/1  "<psi_pm>"
  Bus Selector/6 -> Data Type Conversion7/1  "<L_z1>"
  Bus Selector/7 -> Data Type Conversion8/1  "<L_z2>"
  Bus Selector/11 -> Data Type Conversion12/1  "<L_y2>"
  Bus Selector/3 -> Data Type Conversion4/1  "<R_1>"
  Bus Selector/10 -> Data Type Conversion11/1  "<L_x2>"
  physical_parameters/1 -> Bus Selector/1
  Bus Selector/9 -> Data Type Conversion10/1  "<L_y1>"
  [polepairs] -> Product10/2
  [L_x1] -> Divide5/2
  [L_y1] -> Divide7/2
  [L_x2] -> Divide9/2
  [L_y2] -> Divide11/2
  [L_z3] -> Divide13/2
  Sum/1 -> integrator/1(in)
  Sum1/1 -> integrator1/1(in)
  Add/1 -> integrator2/1(in)
  Add1/1 -> integrator3/1(in)
  Add2/1 -> integrator4/1(in)
  Add3/1 -> integrator5/1(in)
  Add4/1 -> integrator6/1(in)
  Add5/1 -> integrator7/1(in)
  Add6/1 -> integrator8/1(in)
  u_d/1 -> Sum/2
  Data Type Conversion1/1 -> [reciprocal_Ld]
  Data Type Conversion3/1 -> [L_z3]
  Bus Selector/12 -> Data Type Conversion3/1  "<L_z3>"
  Data Type Conversion2/1 -> [reciprocal_Lq]
  Data Type Conversion4/1 -> [R1], Product7/2, Product8/2
  Data Type Conversion5/1 -> [polepairs]
  Data Type Conversion6/1 -> [psi_PM]
  Data Type Conversion7/1 -> [L_z1]
  Data Type Conversion8/1 -> [L_z2]
  Data Type Conversion9/1 -> [L_x1]
  Data Type Conversion10/1 -> [L_y1]
  Data Type Conversion11/1 -> [L_x2]
  Data Type Conversion12/1 -> [L_y2]

== system gm_Copy_of_uz_pmsm_model_9ph_21b_all_double/uz_pmsm_model_9ph/dq_model_9ph/torque_calculation ==
  I_d : Inport
  I_q : Inport  Port=2
  psi_d : Inport  Port=3
  psi_q : Inport  Port=4
  polepairs : Inport  Port=5
  Factor : Gain  Gain=9/2
  Product2 : Product
  Product3 : Product
  Product9 : Product
  Sum3 : Sum  Inputs=-|+
  M_Mi : Outport
  wires:
  Sum3/1 -> Factor/1
  Product3/1 -> Sum3/2
  Product2/1 -> Sum3/1
  psi_q/1 -> Product2/2
  psi_d/1 -> Product3/1
  I_d/1 -> Product2/1
  I_q/1 -> Product3/2
  Product9/1 -> M_Mi/1  "M_Mi"
  polepairs/1 -> Product9/2
  Factor/1 -> Product9/1  "M_Mi"

== system gm_Copy_of_uz_pmsm_model_9ph_21b_all_double/uz_pmsm_model_9ph/dq_model_9ph/mechanical_system/integrator ==
  in : Inport
  reset : Inport  Port=2
  Delay1 : Delay  DelayLength=1  ExternalReset=Level
      settings: InputPortMap=u0,r5
  Gain : Gain  Gain=ts  OutDataTypeStr=Inherit: Same as input
  Sum3 : Sum  Inputs=|++  OutDataTypeStr=Inherit: Same as first input
  outt : Outport
  wires:
  reset/1 -> Delay1/2
  Gain/1 -> Sum3/1
  in/1 -> Gain/1
  Delay1/1 -> outt/1, Sum3/2
  Sum3/1 -> Delay1/1

== system gm_Copy_of_uz_pmsm_model_9ph_21b_all_double/uz_pmsm_model_9ph/dq_model_9ph/pmsm/integrator ==
  in : Inport
  reset : Inport  Port=2
  Delay1 : Delay  DelayLength=1  ExternalReset=Level
      settings: InputPortMap=u0,r5
  Gain : Gain  Gain=ts  OutDataTypeStr=Inherit: Same as input
  Sum3 : Sum  Inputs=|++  OutDataTypeStr=Inherit: Same as first input
  outt : Outport
  wires:
  reset/1 -> Delay1/2
  Gain/1 -> Sum3/1
  in/1 -> Gain/1
  Delay1/1 -> outt/1, Sum3/2
  Sum3/1 -> Delay1/1

== system gm_Copy_of_uz_pmsm_model_9ph_21b_all_double/uz_pmsm_model_9ph/dq_model_9ph/pmsm/integrator1 ==
  in : Inport
  reset : Inport  Port=2
  Delay1 : Delay  DelayLength=1  ExternalReset=Level
      settings: InputPortMap=u0,r5
  Gain : Gain  Gain=ts  OutDataTypeStr=Inherit: Same as input
  Sum3 : Sum  Inputs=|++  OutDataTypeStr=Inherit: Same as first input
  outt : Outport
  wires:
  reset/1 -> Delay1/2
  Gain/1 -> Sum3/1
  in/1 -> Gain/1
  Delay1/1 -> outt/1, Sum3/2
  Sum3/1 -> Delay1/1

== system gm_Copy_of_uz_pmsm_model_9ph_21b_all_double/uz_pmsm_model_9ph/dq_model_9ph/pmsm/integrator2 ==
  in : Inport
  reset : Inport  Port=2
  Delay1 : Delay  DelayLength=1  ExternalReset=Level
      settings: InputPortMap=u0,r5
  Gain : Gain  Gain=ts  OutDataTypeStr=Inherit: Same as input
  Sum3 : Sum  Inputs=|++  OutDataTypeStr=Inherit: Same as first input
  outt : Outport
  wires:
  reset/1 -> Delay1/2
  Gain/1 -> Sum3/1
  in/1 -> Gain/1
  Delay1/1 -> outt/1, Sum3/2
  Sum3/1 -> Delay1/1

== system gm_Copy_of_uz_pmsm_model_9ph_21b_all_double/uz_pmsm_model_9ph/dq_model_9ph/pmsm/integrator3 ==
  in : Inport
  reset : Inport  Port=2
  Delay1 : Delay  DelayLength=1  ExternalReset=Level
      settings: InputPortMap=u0,r5
  Gain : Gain  Gain=ts  OutDataTypeStr=Inherit: Same as input
  Sum3 : Sum  Inputs=|++  OutDataTypeStr=Inherit: Same as first input
  outt : Outport
  wires:
  reset/1 -> Delay1/2
  Gain/1 -> Sum3/1
  in/1 -> Gain/1
  Delay1/1 -> outt/1, Sum3/2
  Sum3/1 -> Delay1/1

== system gm_Copy_of_uz_pmsm_model_9ph_21b_all_double/uz_pmsm_model_9ph/dq_model_9ph/pmsm/integrator4 ==
  in : Inport
  reset : Inport  Port=2
  Delay1 : Delay  DelayLength=1  ExternalReset=Level
      settings: InputPortMap=u0,r5
  Gain : Gain  Gain=ts  OutDataTypeStr=Inherit: Same as input
  Sum3 : Sum  Inputs=|++  OutDataTypeStr=Inherit: Same as first input
  outt : Outport
  wires:
  reset/1 -> Delay1/2
  Gain/1 -> Sum3/1
  in/1 -> Gain/1
  Delay1/1 -> outt/1, Sum3/2
  Sum3/1 -> Delay1/1

== system gm_Copy_of_uz_pmsm_model_9ph_21b_all_double/uz_pmsm_model_9ph/dq_model_9ph/pmsm/integrator5 ==
  in : Inport
  reset : Inport  Port=2
  Delay1 : Delay  DelayLength=1  ExternalReset=Level
      settings: InputPortMap=u0,r5
  Gain : Gain  Gain=ts  OutDataTypeStr=Inherit: Same as input
  Sum3 : Sum  Inputs=|++  OutDataTypeStr=Inherit: Same as first input
  outt : Outport
  wires:
  reset/1 -> Delay1/2
  Gain/1 -> Sum3/1
  in/1 -> Gain/1
  Delay1/1 -> outt/1, Sum3/2
  Sum3/1 -> Delay1/1

== system gm_Copy_of_uz_pmsm_model_9ph_21b_all_double/uz_pmsm_model_9ph/dq_model_9ph/pmsm/integrator6 ==
  in : Inport
  reset : Inport  Port=2
  Delay1 : Delay  DelayLength=1  ExternalReset=Level
      settings: InputPortMap=u0,r5
  Gain : Gain  Gain=ts  OutDataTypeStr=Inherit: Same as input
  Sum3 : Sum  Inputs=|++  OutDataTypeStr=Inherit: Same as first input
  outt : Outport
  wires:
  reset/1 -> Delay1/2
  Gain/1 -> Sum3/1
  in/1 -> Gain/1
  Delay1/1 -> outt/1, Sum3/2
  Sum3/1 -> Delay1/1

== system gm_Copy_of_uz_pmsm_model_9ph_21b_all_double/uz_pmsm_model_9ph/dq_model_9ph/pmsm/integrator7 ==
  in : Inport
  reset : Inport  Port=2
  Delay1 : Delay  DelayLength=1  ExternalReset=Level
      settings: InputPortMap=u0,r5
  Gain : Gain  Gain=ts  OutDataTypeStr=Inherit: Same as input
  Sum3 : Sum  Inputs=|++  OutDataTypeStr=Inherit: Same as first input
  outt : Outport
  wires:
  reset/1 -> Delay1/2
  Gain/1 -> Sum3/1
  in/1 -> Gain/1
  Delay1/1 -> outt/1, Sum3/2
  Sum3/1 -> Delay1/1

== system gm_Copy_of_uz_pmsm_model_9ph_21b_all_double/uz_pmsm_model_9ph/dq_model_9ph/pmsm/integrator8 ==
  in : Inport
  reset : Inport  Port=2
  Delay1 : Delay  DelayLength=1  ExternalReset=Level
      settings: InputPortMap=u0,r5
  Gain : Gain  Gain=ts  OutDataTypeStr=Inherit: Same as input
  Sum3 : Sum  Inputs=|++  OutDataTypeStr=Inherit: Same as first input
  outt : Outport
  wires:
  reset/1 -> Delay1/2
  Gain/1 -> Sum3/1
  in/1 -> Gain/1
  Delay1/1 -> outt/1, Sum3/2
  Sum3/1 -> Delay1/1
